simulink library "satAttDcmPDController_sl"  (R2023b)
settings: Solver=VariableStepAuto  StartTime=0.0  StopTime=10.0  RelTol=1e-3
undefined symbols (not defined in the file): innerAngDistGain, kD, kP, maxGimbalRate, outerAngDistGain, rotorAngRate, rotorInertia
libraries: magnetometerSensorHW_sl x1
settings Model: Creator=gilbu  LastModifiedBy=gilbu

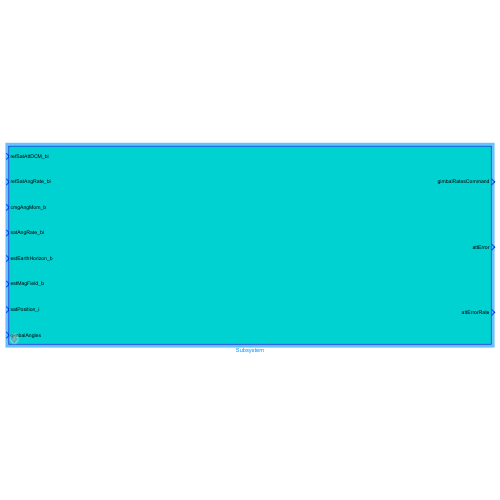
[thumbnail: Simulink's stored preview of the top-level diagram]
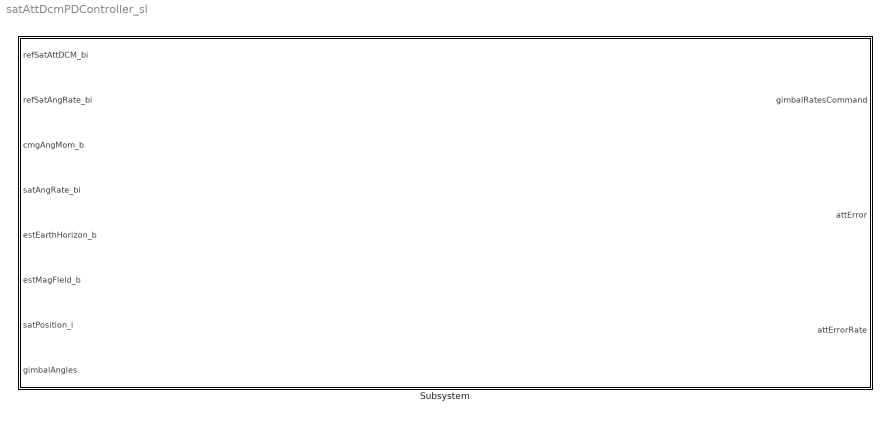
== system satAttDcmPDController_sl ==
  Subsystem : Subsystem  mask{kP=kP, kD=kD, rotorInertia=rotorInertia, rotorAngRate=rotorAngRate, maxGimbalRate=maxGimbalRate, innerAngDistGain=innerAngDistGain, outerAngDistGain=outerAngDistGain, satInertiaTensor=0}
      mask prompts: kP "Proportional Gain Vector <3> [-]"; kD "Derivatie Gain Vector <3> [-]"; rotorInertia "Rotor Wheel Moment of Inertia <1> [kgm2]"; rotorAngRate "Rotor Wheel angular rate <1> [rad/s]"; maxGimbalRate "Max Gimbal Rate <1> [rad/s}"; innerAngDistGain "Inner Gimbal Angle Distribution Gain <1> [-]"; outerAngDistGain "Outer Gimbal Angle Distribution Gain <1> [-]"; satInertiaTensor "Satellite Inertia Tensor <3,3> [kg*m2]"
      mask DialogControl DescTextVar Prompt: Earth Point Attitude Determinatin and PD Controller based on Attitude DCM error, and angualr rate error for satellite with rigid body dynamics in ciruclar orbit. Includes Steering law for four parallel mounted DGCMGs.
      mask DialogControl Control2 Prompt: Attitude Determination used TRIAD algorithm and mesurements from magnetometer and Earth Horizon Sensors.

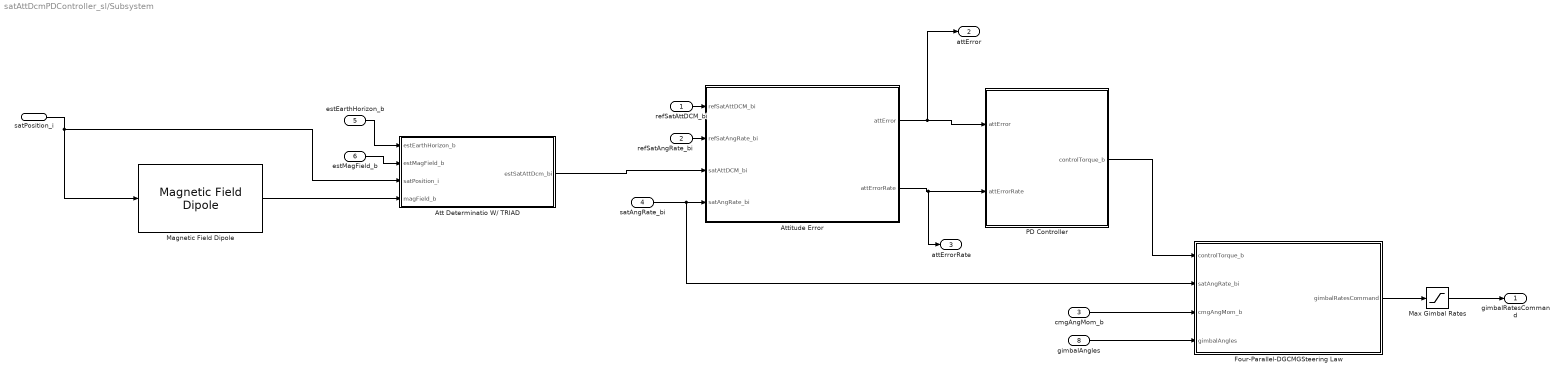
== system satAttDcmPDController_sl/Subsystem ==
  refSatAttDCM_bi : Inport
  refSatAngRate_bi : Inport  Port=2
  cmgAngMom_b : Inport  Port=3
  satAngRate_bi : Inport  Port=4
  estEarthHorizon_b : Inport  Port=5
  estMagField_b : Inport  Port=6
  satPosition_i : Inport  Port=7
  gimbalAngles : Inport  Port=8
  Att Determinatio W/ TRIAD : MATLAB Function  TreatAsAtomicUnit=on
  Attitude Error : MATLAB Function  TreatAsAtomicUnit=on
  Four-Parallel-DGCMGSteering Law : MATLAB Function  TreatAsAtomicUnit=on
  Magnetic Field Dipole : magnetometerSensorHW_sl/Magnetometer Measurments/Magnetic Field Dipole  SystemSampleTime=-1  VariantActivationTime=update diagram  AllowFlexibleInterface=on  Latency=0  AutoFrameSizeCalculation=off
  Max Gimbal Rates : Saturate  UpperLimit=maxGimbalRate  LowerLimit=-maxGimbalRate  ZeroCross=off
  PD Controller : MATLAB Function  TreatAsAtomicUnit=on
  gimbalRatesCommand : Outport
  attError : Outport  Port=2
  attErrorRate : Outport  Port=3
  wires:
  PD Controller/1(controlTorque_b) -> Four-Parallel-DGCMGSteering Law/1(controlTorque_b)
  Attitude Error/2(attErrorRate) -> attErrorRate/1, PD Controller/2(attErrorRate)
  Attitude Error/1(attError) -> attError/1, PD Controller/1(attError)
  satAngRate_bi/1 -> Four-Parallel-DGCMGSteering Law/2(satAngRate_bi), Attitude Error/4(satAngRate_bi)
  refSatAttDCM_bi/1 -> Attitude Error/1(refSatAttDCM_bi)
  refSatAngRate_bi/1 -> Attitude Error/2(refSatAngRate_bi)
  Four-Parallel-DGCMGSteering Law/1(gimbalRatesCommand) -> Max Gimbal Rates/1
  cmgAngMom_b/1 -> Four-Parallel-DGCMGSteering Law/3(cmgAngMom_b)
  Att Determinatio W/ TRIAD/1(estSatAttDcm_bi) -> Attitude Error/3(satAttDCM_bi)
  estEarthHorizon_b/1 -> Att Determinatio W/ TRIAD/1(estEarthHorizon_b)
  estMagField_b/1 -> Att Determinatio W/ TRIAD/2(estMagField_b)
  satPosition_i/1 -> Magnetic Field Dipole/1, Att Determinatio W/ TRIAD/3(satPosition_i)
  Magnetic Field Dipole/1 -> Att Determinatio W/ TRIAD/4(magField_b)
  gimbalAngles/1 -> Four-Parallel-DGCMGSteering Law/4(gimbalAngles)
  Max Gimbal Rates/1 -> gimbalRatesCommand/1

== matlab function satAttDcmPDController_sl/Subsystem/PD Controller ==
  data: attError input size=3; controlTorque_b output size=3; attErrorRate input size=3; kP parameter size=3; kD parameter size=3; satInertiaTensor parameter size=3,3
function controlTorque_b = satAttPDControl( ...
    attError,attErrorRate, ... % Error Inputs
    kP, kD, satInertiaTensor)... % Parameters
%-------------------------------------------------------------------------------
% Construct Gain Matrices

KP = diag(kP);
KD = diag(kD);


%-------------------------------------------------------------------------------
% Calcualte control input U
u = KP*attError+KD*attErrorRate;
controlTorque_b = satInertiaTensor*u;
%-------------------------------------------------------------------------------
end

== matlab function satAttDcmPDController_sl/Subsystem/Attitude Error ==
  data: refSatAttDCM_bi input size=3,3; refSatAngRate_bi input size=3; attError output size=3; satAttDCM_bi input size=3,3; satAngRate_bi input size=3; attErrorRate output size=3
function [attError,attErrorRate]=attError( ...
    refSatAttDCM_bi,refSatAngRate_bi, ...% Reference State inputs ...
    satAttDCM_bi,satAngRate_bi... % Actual State Input
    )
%-------------------------------------------------------------------------------
% Construct angular rate skew symmetric matrix
omegaSkew = [0 -refSatAngRate_bi(3) refSatAngRate_bi(2);
             refSatAngRate_bi(3) 0 -refSatAngRate_bi(1);
             -refSatAngRate_bi(2) refSatAngRate_bi(1) 0 ];
%-------------------------------------------------------------------------------
% Rate and Quaternion Error Calculation

%DCM Error
dcmDelta = satAttDCM_bi*refSatAttDCM_bi';

% Angular Rate Error
deltaSatAngRate = satAngRate_bi-refSatAngRate_bi;

%-------------------------------------------------------------------------------
% Attitude Error Calculations

% Error
attError = -0.5.*[dcmDelta(3,2)-dcmDelta(2,3);
                dcmDelta(1,3)-dcmDelta(3,1);
                dcmDelta(2,1)-dcmDelta(1,2)];
% Error Rate
attErrorRate = -omegaSkew*attError+deltaSatAngRate;
end

%-------------------------------------------------------------------------------

== matlab function satAttDcmPDController_sl/Subsystem/Four-Parallel-DGCMGSteering Law ==
  data: controlTorque_b input size=3; gimbalRatesCommand output size=8; satAngRate_bi input size=3; cmgAngMom_b input size=3; gimbalAngles input size=8; rotorInertia parameter size=1; innerAngDistGain parameter size=1; outerAngDistGain parameter size=1; rotorAngRate parameter size=1
function gimbalRatesCommand = dgcmgSteeringLaw( ...
    controlTorque_b,satAngRate_bi,cmgAngMom_b,gimbalAngles,... %Inputs
    rotorInertia,innerAngDistGain,outerAngDistGain,... % Parameters
      rotorAngRate)
%-------------------------------------------------------------------------------
% Initialize Variables

% Commanded Gimbal Rates
gimbalRatesCommand = zeros(8,1);

% Inner and Outer Gimbal Angles
innerAng = gimbalAngles(1:2:8);
outerAng = gimbalAngles(2:2:8);

% Rotor Angular Momentum
rotorAngMom = rotorInertia*rotorAngRate;

% Trig Functions
sa1 = sin(gimbalAngles(1));
ca1 = cos(gimbalAngles(1));
cb1 = cos(gimbalAngles(2));
sb1 = sin(gimbalAngles(2));

sa2 = sin(gimbalAngles(3));
ca2 = cos(gimbalAngles(3));
cb2 = cos(gimbalAngles(4));
sb2 = sin(gimbalAngles(4));

sa3 = sin(gimbalAngles(5));
ca3 = cos(gimbalAngles(5));
cb3 = cos(gimbalAngles(6));
sb3 = sin(gimbalAngles(6));

sa4 = sin(gimbalAngles(7));
ca4 = cos(gimbalAngles(7));
cb4 = cos(gimbalAngles(8));
sb4 = sin(gimbalAngles(8));

cAlpha = [ca1 ca2 ca3 ca4];
cBeta = [cb1 cb2 cb3 cb4];
sAlpha = [sa1 sa2 sa3 sa4];
sBeta = [sb1 sb2 sb3 sb4];

% Gimbal Direction Matrix
C = [sa1 sa2 sa3 sa4;
     cb1*ca1 cb1*ca2 cb3*ca3 cb4*ca4;
     sb1*ca1 sb2*ca2 sb3*ca3 sb4*ca4];

% Construct angular rate skew symmetric matrix
omegaSkew = [0 -satAngRate_bi(3) satAngRate_bi(2);
             satAngRate_bi(3) 0 -satAngRate_bi(1);
             -satAngRate_bi(2) satAngRate_bi(1) 0 ];

% Construct B  and C Matrix for Outer gimbal psuedo-inverse
b1 = -rotorAngMom.*cAlpha(:).*sBeta(:);
b2 = rotorAngMom.*cAlpha(:).*cBeta(:);

bMat = [b1'; b2'];
c11 = b1'*b1;
c22 = b2'*b2;
c12 = b1'*b2;
cMat =inv([c11 c12;c12 c22]+1e-6.*eye(2));

% Outer Gimbal Distribution
betaDotDist = zeros(4,1);

%-------------------------------------------------------------------------------
% Reactino Wheel Command

% Desired Control Torque.
u = -controlTorque_b-omegaSkew*cmgAngMom_b;

%----------------------------------------
% Kennels DGCMG Steering Law

% Desired inner gimbal angles alpha_i
hca = rotorAngMom.*cAlpha(:);
hcaSum = sum(hca);
hcaa = hca(:).*innerAng(:);
alphaStar =sum(hcaa)./hcaSum;

innerRateCommand = zeros(4,1);
for i = 1:4
innerRateCommand(i) = u(1)/hcaSum+innerAngDistGain*(alphaStar-innerAng(i));
end


% Outer Gimbal Rate Distribution based on CMG pair repulsion.

for i = 1:4
    betaDot = zeros(1,4);
    for j = 1:4
        
        if i==j
            deltaij = 1;
        else 
            deltaij = 0;
        end

        betaDot(j) = (rotorAngMom^2.*(outerAng(i)-outerAng(j)-pi.*sign(outerAng(i)-outerAng(j)))).*(1-deltaij);
        
    end
    betaDotDist(i) = -outerAngDistGain*sum(betaDot);
    % betaDotDist(i) =  max(betaDotDist(i),-.2);
    % betaDotDist(i) = min(betaDotDist(i),.2);
end

% Outer Gimbal Torque
torque2 = rotorAngMom.*(cAlpha(:).*sBeta(:).*betaDotDist(:) + sAlpha(:).*cBeta(:).*innerRateCommand(:)) ;
torque3 = rotorAngMom.*(-cAlpha(:).*cBeta(:).*betaDotDist(:) + sAlpha(:).*sBeta(:).*innerRateCommand(:));
torque23 = [sum(torque2); sum(torque3)];

modCommandTorque = [u(2); u(3);]+torque23;

% Robust Psuedo Inverse
% lambda = 1e-12;
% bMatDagger = bMat'/(bMat*bMat'+lambda*eye(2));

outerRateCommand = bMat'*cMat*modCommandTorque+betaDotDist;

% Assing gimbal rates accordingly
gimbalRatesCommand(1:2:8) = innerRateCommand;
gimbalRatesCommand(2:2:8) = outerRateCommand;


%-------------------------------------------------------------------------------
end

== matlab function satAttDcmPDController_sl/Subsystem/Att Determinatio W// TRIAD ==
  data: estSatAttDcm_bi output size=3,3; estEarthHorizon_b input size=3; estMagField_b input size=3; satPosition_i input size=3; magField_b input size=3
function estSatAttDcm_bi = triadAttDet( ...
    estEarthHorizon_b,estMagField_b,satPosition_i,magField_b... % Inputs
    ... % Parameters
    )
%-------------------------------------------------------------------------------
% Initialize direction Vecotrs

% Earth horizon direction measurement d_b1
d_b1 = estEarthHorizon_b./norm(estEarthHorizon_b);

%Known earth horizon directio d_i1
d_i1 = satPosition_i./norm(satPosition_i);

% Magnetometer directon measruemtn d_b2
d_b2 = estMagField_b./norm(estMagField_b);

% Known magnetic field direction d_b1
d_i2 = magField_b./norm(magField_b);


% ------------------------------------------------------------------------------
% TRIAD Algorithm

% Body Directions
t_bx = d_b1;

b1b2Cross = cross(d_b1,d_b2);
t_bz = b1b2Cross./norm(b1b2Cross);

t_by = cross(t_bz,t_bx);

% Inertial Direction
t_ix = d_i1;

i1i2Cross = cross(d_i1,d_i2);
t_iz =i1i2Cross./norm(i1i2Cross);

t_iy = cross(t_ix,t_iz);

% Construct Estimated DCM

estSatAttDcm_bi = [t_bx t_by t_bz]*[t_ix t_iy t_iz]';


%-------------------------------------------------------------------------------
end
